simulink model "sys_sim"  (R2021a)
settings: Solver=VariableStepAuto  StartTime=0.0  StopTime=10.0  RelTol=1e-3
settings Model: Creator=Suman  LastModifiedBy=Suman

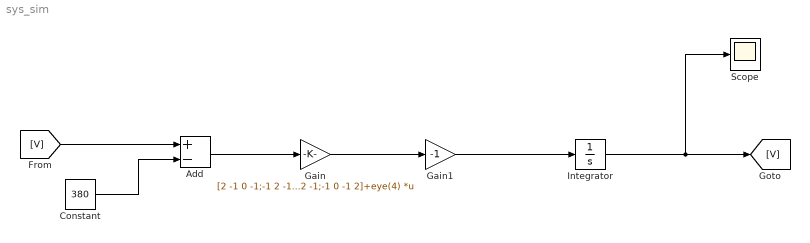
== system sys_sim ==
  Add : Sum  Inputs=+-
  Constant : Constant  Value=380
  Gain : Gain  Gain=[2 -1 0 -1;-1 2 -1 0;0 -1 2 -1;-1 0 -1 2]+eye(4)  Multiplication=Matrix(K*u) (u vector)
  Gain1 : Gain  Gain=-1
  Integrator : Integrator  InitialCondition="[287.1501 ; 145.6127 ; 240.0841 ;  42.5659]"
  Scope : Scope
  wires:
  Gain/1 -> Gain1/1
  Gain1/1 -> Integrator/1
  Integrator/1 -> Scope/1, [V]
  Add/1 -> Gain/1
  [V] -> Add/1
  Constant/1 -> Add/2
